simulink model "gm_IP_Core_SS_Switch_and_PWM"  (R2021a)
settings: Solver=VariableStepAuto  StartTime=0.0  StopTime=0.0002  RelTol=1e-3
undefined symbols (not defined in the file or in its folder): f_FPGA_clk, T_FPGA_clk
libraries: hdlmdlgenlib x3, hdlsllib x3
(part 1 of 2)
settings Model: Creator=BHK  LastModifiedBy=hufnagelde
settings SolverCC: AlgebraicLoopSolver=TrustRegion
settings DataIOCC: ReturnWorkspaceOutputs=off
settings OptimizationCC: BlockReduction=off  ConditionallyExecuteInputs=off  DefaultParameterBehavior=Inlined
settings DebuggingCC: AlgebraicLoopMsg=error  InheritedTsInSrcMsg=none  SFMachineParentedDataDiag=warning  ArithmeticOperatorsInVariantConditions=warning
settings HardwareCC: ProdBitPerPointer=32  ProdBitPerSizeT=32  ProdBitPerPtrDiffT=32  ProdLargestAtomicFloat=None  ProdIntDivRoundTo=Undefined  ProdEndianess=Unspecified  ProdWordSize=32  ProdHWDeviceType=ASIC/FPGA->ASIC/FPGA  TargetBitPerLong=64  TargetBitPerPointer=64  TargetBitPerSizeT=64  TargetBitPerPtrDiffT=64  TargetLongLongMode=on  TargetIntDivRoundTo=Zero  TargetEndianess=LittleEndian  TargetWordSize=64  TargetHWDeviceType=Custom Processor->MATLAB Host Computer  ProdEqTarget=off
settings SFSimCC: SimUseLocalCustomCode=off  CustomCodeUndefinedFunction=UseInterfaceOnly
settings RTWCC: RTWUseLocalCustomCode=off

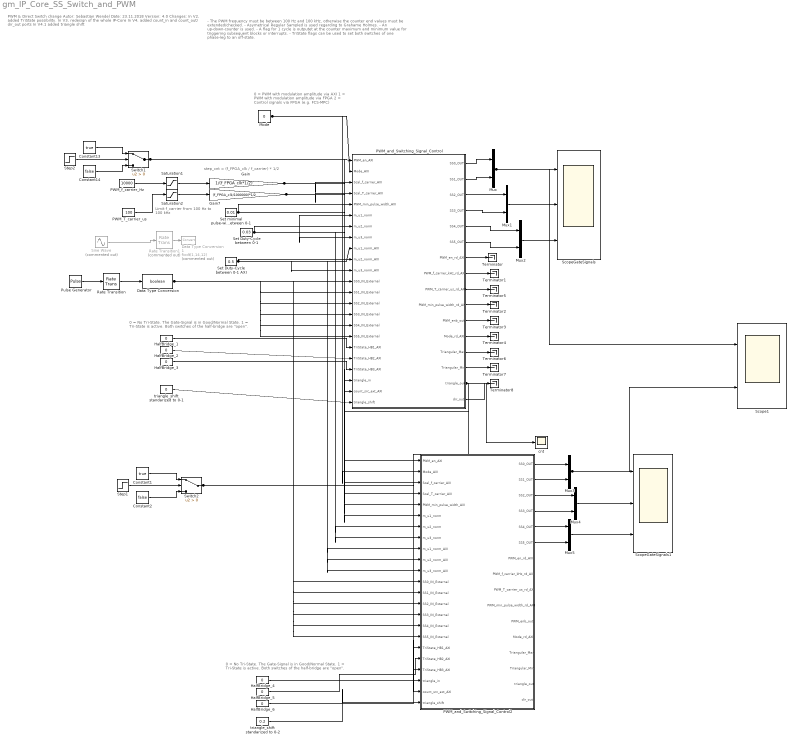
== system gm_IP_Core_SS_Switch_and_PWM ==
  note: 0 = No Tri-State. The Gate-Signal is in Good/Normal State.
      | 1 = Tri-State is active. Both switches of the half-bridge are "open".
  note: - The PWM frequency must be between 100 Hz and 100 kHz, otherwise the counter end values must be extended/checked.
      | - Asymetrical Regular Sampled is used regarding to Grahame Holmes.
      | - An up-down-counter is used.
      | - A flag for 1 cycle is outputet at the counter maximum and minimum value for triggering subsequent blocks or interrupts.
      | - TriState flags can be used to set both switches of one phase-leg to an off-state.
  note: Limit f_carrier from
      | 100 Hz to 100 kHz
  note: step_cnt = (f_FPGA_clk / f_carrier) * 1/2
  note: 0 = PWM with modulation amplitude via AXI
      | 1 = PWM with modulation amplitude via FPGA
      | 2 = Control signals via FPGA (e.g. FCS-MPC)
  note: PWM & Direct Switch change
      |
      | Autor: Sebastian Wendel
      | Date: 23.11.2018
      | Version: 4.0
      | Changes: In V2, added TriState possibility.
      | In V3, redesign of the whole IP-Core
      | In V4, added count_in and count_out/
      | dir_out ports
      | In V4.1 added triangle shift
  note: 0 = No Tri-State. The Gate-Signal is in Good/Normal State.
      | 1 = Tri-State is active. Both switches of the half-bridge are "open".
  Constant1 : Constant  Value=true  SampleTime=T_FPGA_clk
  Constant13 : Constant  Value=true  SampleTime=T_FPGA_clk
  Constant14 : Constant  Value=false  SampleTime=T_FPGA_clk
  Constant2 : Constant  Value=false  SampleTime=T_FPGA_clk
  Data Type Conversion : DataTypeConversion  OutDataTypeStr=boolean
  Data Type Conversion1 : DataTypeConversion  Commented=on  OutDataTypeStr=fixdt(1,14,12)
  Gain : Gain  Gain=1/(f_FPGA_clk*1/2)  OutDataTypeStr=fixdt(0,25,26)
  Gain7 : Gain  Gain=(f_FPGA_clk/1000000)*1/2  OutDataTypeStr=fixdt(0,25,0)
  HalfBridge_{1..6} (6 alike) : Constant  Value=0  OutDataTypeStr=fixdt(0,2,0)  SampleTime=T_FPGA_clk
  Mode : Constant  Value=0  OutDataTypeStr=fixdt(0,2,0)  SampleTime=T_FPGA_clk
  Mux{,1..5} (6 alike) : Mux  Inputs=2
  PWM_T_carrier_us : Constant  Value=100  OutDataTypeStr=uint32  SampleTime=T_FPGA_clk
  PWM_and_Switching_Signal_Control : Subsystem  TreatAsAtomicUnit=on
  PWM_and_Switching_Signal_Control2 : Subsystem  TreatAsAtomicUnit=on
  PWM_f_carrier_Hz : Constant  Value=10000  OutDataTypeStr=uint32  SampleTime=T_FPGA_clk
  Pulse Generator : DiscretePulseGenerator  PulseType=Time based  Period=0.01  PulseWidth=5
  Rate Transition : RateTransition  OutPortSampleTime=T_FPGA_clk
  Rate Transition1 : RateTransition  Commented=on  OutPortSampleTime=T_FPGA_clk
  Saturation1 : Saturate  UpperLimit=100000  LowerLimit=100
  Saturation2 : Saturate  UpperLimit=10000  LowerLimit=10
  Scope1 : Scope  NumInputPorts=2
  ScopeGateSignals : Scope  NumInputPorts=3
  ScopeGateSignals1 : Scope  NumInputPorts=3
  Set Duty-Cycle between 0-1 : Constant  Value=0.03  OutDataTypeStr=fixdt(1,14,12)  SampleTime=T_FPGA_clk
  Set Duty-Cycle between 0-1 AXI : Constant  Value=0.5  OutDataTypeStr=fixdt(1,14,12)  SampleTime=T_FPGA_clk
  Set minimal pulse-width between 0-1 : Constant  Value=0.01  OutDataTypeStr=fixdt(1,18,16)  SampleTime=T_FPGA_clk
  Sine Wave : Sin  Commented=on  Frequency=500  SampleTime=0
  Step1 : Step  Time=0.002  Before=1  SampleTime=T_FPGA_clk
  Step2 : Step  Time=0.002  Before=1  SampleTime=T_FPGA_clk
  Switch1 : Switch  Criteria=u2 > Threshold
  Switch2 : Switch  Criteria=u2 > Threshold
  Terminator{,1..8} (9 alike) : Terminator
  cnt : Scope
  triangle_shift standarized to 0-1 : Constant  Value=0  OutDataTypeStr=fixdt(0,18,17)  SampleTime=T_FPGA_clk
  triangle_shift standarized to 0-2 : Constant  Value=0.2  OutDataTypeStr=fixdt(0,18,17)  SampleTime=T_FPGA_clk
  wires:
  triangle_shift standarized to 0-2/1 -> PWM_and_Switching_Signal_Control2/23(triangle_shift)
  triangle_shift standarized to 0-1/1 -> PWM_and_Switching_Signal_Control/23(triangle_shift)
  Mux4/1 -> ScopeGateSignals1/2
  PWM_and_Switching_Signal_Control2/6(SS5_OUT) -> Mux5/2
  PWM_and_Switching_Signal_Control2/4(SS3_OUT) -> Mux4/2
  PWM_and_Switching_Signal_Control2/3(SS2_OUT) -> Mux4/1
  PWM_and_Switching_Signal_Control2/5(SS4_OUT) -> Mux5/1
  Mux5/1 -> ScopeGateSignals1/3
  Mux3/1 -> Scope1/2, ScopeGateSignals1/1
  PWM_and_Switching_Signal_Control2/2(SS1_OUT) -> Mux3/2
  PWM_and_Switching_Signal_Control2/1(SS0_OUT) -> Mux3/1
  HalfBridge_5/1 -> PWM_and_Switching_Signal_Control2/19(TriState_HB2_AXI)
  HalfBridge_6/1 -> PWM_and_Switching_Signal_Control2/20(TriState_HB3_AXI)
  HalfBridge_4/1 -> PWM_and_Switching_Signal_Control2/18(TriState_HB1_AXI)
  Data Type Conversion/1 -> PWM_and_Switching_Signal_Control/12(SS0_IN_External), PWM_and_Switching_Signal_Control/13(SS1_IN_External), PWM_and_Switching_Signal_Control/14(SS2_IN_External), PWM_and_Switching_Signal_Control/15(SS3_IN_External), PWM_and_Switching_Signal_Control/16(SS4_IN_External), PWM_and_Switching_Signal_Control/17(SS5_IN_External), PWM_and_Switching_Signal_Control2/12(SS0_IN_External), PWM_and_Switching_Signal_Control2/13(SS1_IN_External), PWM_and_Switching_Signal_Control2/15(SS3_IN_External), PWM_and_Switching_Signal_Control2/17(SS5_IN_External), PWM_and_Switching_Signal_Control2/16(SS4_IN_External), PWM_and_Switching_Signal_Control2/14(SS2_IN_External)
  PWM_and_Switching_Signal_Control/15(triangle_out) -> PWM_and_Switching_Signal_Control/21(triangle_in), PWM_and_Switching_Signal_Control2/21(triangle_in), cnt/1
  Switch2/1 -> PWM_and_Switching_Signal_Control/22(count_src_ext_AXI), PWM_and_Switching_Signal_Control2/22(count_src_ext_AXI)
  Constant1/1 -> Switch2/1
  Step1/1 -> Switch2/2
  Constant2/1 -> Switch2/3
  PWM_and_Switching_Signal_Control/16(dir_out) -> Terminator8/1
  Set Duty-Cycle between 0-1/1 -> PWM_and_Switching_Signal_Control2/6(m_u1_norm), PWM_and_Switching_Signal_Control2/7(m_u2_norm), PWM_and_Switching_Signal_Control2/8(m_u3_norm), PWM_and_Switching_Signal_Control/7(m_u2_norm), PWM_and_Switching_Signal_Control/8(m_u3_norm), PWM_and_Switching_Signal_Control/6(m_u1_norm)
  Rate Transition1/1 -> Data Type Conversion1/1
  Saturation2/1 -> Gain7/1
  Saturation1/1 -> Gain/1
  Gain7/1 -> PWM_and_Switching_Signal_Control/4(Scal_T_carrier_AXI), PWM_and_Switching_Signal_Control2/4(Scal_T_carrier_AXI)
  Gain/1 -> PWM_and_Switching_Signal_Control2/3(Scal_f_carrier_AXI), PWM_and_Switching_Signal_Control/3(Scal_f_carrier_AXI)
  PWM_and_Switching_Signal_Control/14(Triangular_Min) -> Terminator7/1
  HalfBridge_1/1 -> PWM_and_Switching_Signal_Control/18(TriState_HB1_AXI)
  HalfBridge_2/1 -> PWM_and_Switching_Signal_Control/19(TriState_HB2_AXI)
  HalfBridge_3/1 -> PWM_and_Switching_Signal_Control/20(TriState_HB3_AXI)
  PWM_and_Switching_Signal_Control/13(Triangular_Max) -> Terminator6/1
  PWM_and_Switching_Signal_Control/9(PWM_T_carrier_us_rd_AXI) -> Terminator5/1
  Pulse Generator/1 -> Rate Transition/1
  Rate Transition/1 -> Data Type Conversion/1
  PWM_T_carrier_us/1 -> Saturation2/1
  Mux1/1 -> ScopeGateSignals/2
  Mux2/1 -> ScopeGateSignals/3
  PWM_and_Switching_Signal_Control/6(SS5_OUT) -> Mux2/2
  PWM_and_Switching_Signal_Control/5(SS4_OUT) -> Mux2/1
  PWM_and_Switching_Signal_Control/4(SS3_OUT) -> Mux1/2
  PWM_and_Switching_Signal_Control/3(SS2_OUT) -> Mux1/1
  Mux/1 -> ScopeGateSignals/1, Scope1/1
  PWM_and_Switching_Signal_Control/2(SS1_OUT) -> Mux/2
  PWM_and_Switching_Signal_Control/1(SS0_OUT) -> Mux/1
  Set Duty-Cycle between 0-1 AXI/1 -> PWM_and_Switching_Signal_Control/9(m_u1_norm_AXI), PWM_and_Switching_Signal_Control/10(m_u2_norm_AXI), PWM_and_Switching_Signal_Control/11(m_u3_norm_AXI), PWM_and_Switching_Signal_Control2/11(m_u3_norm_AXI), PWM_and_Switching_Signal_Control2/10(m_u2_norm_AXI), PWM_and_Switching_Signal_Control2/9(m_u1_norm_AXI)
  PWM_and_Switching_Signal_Control/12(Mode_rd_AXI) -> Terminator4/1
  PWM_and_Switching_Signal_Control/11(PWM_enb_out) -> Terminator3/1
  PWM_and_Switching_Signal_Control/10(PWM_min_pulse_width_rd_AXI) -> Terminator2/1
  PWM_and_Switching_Signal_Control/8(PWM_f_carrier_kHz_rd_AXI) -> Terminator1/1
  PWM_and_Switching_Signal_Control/7(PWM_en_rd_AXI) -> Terminator/1
  Sine Wave/1 -> Rate Transition1/1
  Set minimal pulse-width between 0-1/1 -> PWM_and_Switching_Signal_Control2/5(PWM_min_pulse_width_AXI), PWM_and_Switching_Signal_Control/5(PWM_min_pulse_width_AXI)
  PWM_f_carrier_Hz/1 -> Saturation1/1
  Mode/1 -> PWM_and_Switching_Signal_Control/2(Mode_AXI), PWM_and_Switching_Signal_Control2/2(Mode_AXI)
  Switch1/1 -> PWM_and_Switching_Signal_Control2/1(PWM_en_AXI), PWM_and_Switching_Signal_Control/1(PWM_en_AXI)
  Constant14/1 -> Switch1/3
  Constant13/1 -> Switch1/1
  Step2/1 -> Switch1/2

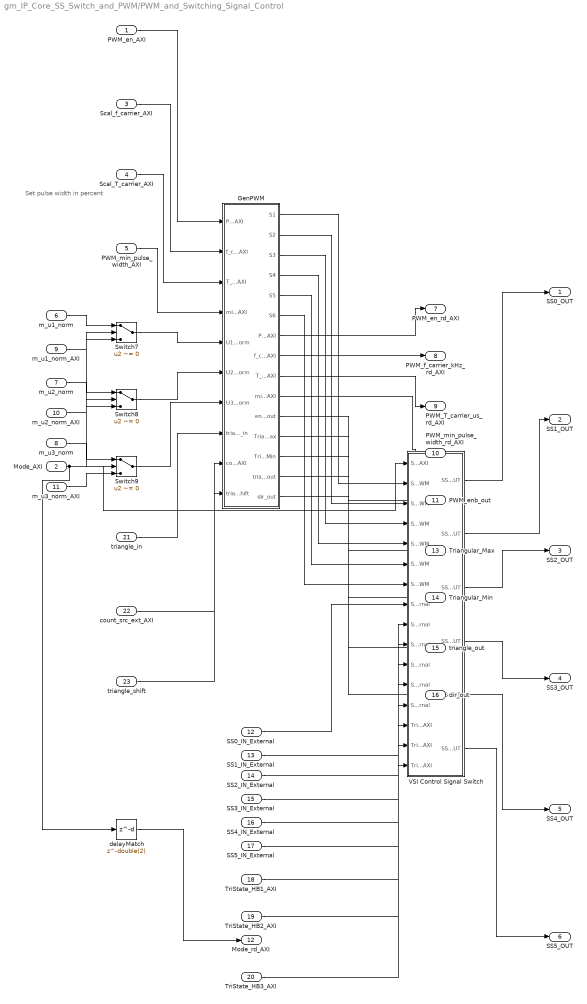
== system gm_IP_Core_SS_Switch_and_PWM/PWM_and_Switching_Signal_Control ==
  note: Set pulse width in percent
  PWM_en_AXI : Inport  OutDataTypeStr=boolean  PortDimensions=1  SampleTime=1e-08
  Mode_AXI : Inport  Port=2  OutDataTypeStr=fixdt(0, 2, 0)  PortDimensions=1  SampleTime=1e-08
  Scal_f_carrier_AXI : Inport  Port=3  OutDataTypeStr=fixdt(0, 25, 26)  PortDimensions=1  SampleTime=1e-08
  Scal_T_carrier_AXI : Inport  Port=4  OutDataTypeStr=fixdt(0, 25, 0)  PortDimensions=1  SampleTime=1e-08
  PWM_min_pulse_width_AXI : Inport  Port=5  OutDataTypeStr=fixdt(1, 18, 16)  PortDimensions=1  SampleTime=1e-08
  m_u1_norm : Inport  Port=6  OutDataTypeStr=fixdt(1, 14, 12)  PortDimensions=1  SampleTime=1e-08
  m_u2_norm : Inport  Port=7  OutDataTypeStr=fixdt(1, 14, 12)  PortDimensions=1  SampleTime=1e-08
  m_u3_norm : Inport  Port=8  OutDataTypeStr=fixdt(1, 14, 12)  PortDimensions=1  SampleTime=1e-08
  m_u1_norm_AXI : Inport  Port=9  OutDataTypeStr=fixdt(1, 14, 12)  PortDimensions=1  SampleTime=1e-08
  m_u2_norm_AXI : Inport  Port=10  OutDataTypeStr=fixdt(1, 14, 12)  PortDimensions=1  SampleTime=1e-08
  m_u3_norm_AXI : Inport  Port=11  OutDataTypeStr=fixdt(1, 14, 12)  PortDimensions=1  SampleTime=1e-08
  SS0_IN_External : Inport  Port=12  OutDataTypeStr=boolean  PortDimensions=1  SampleTime=1e-08
  SS1_IN_External : Inport  Port=13  OutDataTypeStr=boolean  PortDimensions=1  SampleTime=1e-08
  SS2_IN_External : Inport  Port=14  OutDataTypeStr=boolean  PortDimensions=1  SampleTime=1e-08
  SS3_IN_External : Inport  Port=15  OutDataTypeStr=boolean  PortDimensions=1  SampleTime=1e-08
  SS4_IN_External : Inport  Port=16  OutDataTypeStr=boolean  PortDimensions=1  SampleTime=1e-08
  SS5_IN_External : Inport  Port=17  OutDataTypeStr=boolean  PortDimensions=1  SampleTime=1e-08
  TriState_HB1_AXI : Inport  Port=18  OutDataTypeStr=fixdt(0, 2, 0)  PortDimensions=1  SampleTime=1e-08
  TriState_HB2_AXI : Inport  Port=19  OutDataTypeStr=fixdt(0, 2, 0)  PortDimensions=1  SampleTime=1e-08
  TriState_HB3_AXI : Inport  Port=20  OutDataTypeStr=fixdt(0, 2, 0)  PortDimensions=1  SampleTime=1e-08
  triangle_in : Inport  Port=21  OutDataTypeStr=fixdt(0, 18, 17)  PortDimensions=1  SampleTime=1e-08
  count_src_ext_AXI : Inport  Port=22  OutDataTypeStr=boolean  PortDimensions=1  SampleTime=1e-08
  triangle_shift : Inport  Port=23  OutDataTypeStr=fixdt(0, 18, 17)  PortDimensions=1  SampleTime=1e-08
  GenPWM : Subsystem
  Switch7 : Switch  Criteria=u2 ~= 0  Threshold=double(0)  OutDataTypeStr=fixdt(1, 14, 12)  SampleTime=1e-08
  Switch8 : Switch  Criteria=u2 ~= 0  Threshold=double(0)  OutDataTypeStr=fixdt(1, 14, 12)  SampleTime=1e-08
  Switch9 : Switch  Criteria=u2 ~= 0  Threshold=double(0)  OutDataTypeStr=fixdt(1, 14, 12)  SampleTime=1e-08
  VSI Control Signal Switch : Subsystem
  delayMatch : Delay  DelayLength=double(2)  InitialCondition=0  SampleTime=1e-08
  SS0_OUT : Outport  SampleTime=1e-08  VectorParamsAs1DForOutWhenUnconnected=off
  SS1_OUT : Outport  Port=2  SampleTime=1e-08  VectorParamsAs1DForOutWhenUnconnected=off
  SS2_OUT : Outport  Port=3  SampleTime=1e-08  VectorParamsAs1DForOutWhenUnconnected=off
  SS3_OUT : Outport  Port=4  SampleTime=1e-08  VectorParamsAs1DForOutWhenUnconnected=off
  SS4_OUT : Outport  Port=5  SampleTime=1e-08  VectorParamsAs1DForOutWhenUnconnected=off
  SS5_OUT : Outport  Port=6  SampleTime=1e-08  VectorParamsAs1DForOutWhenUnconnected=off
  PWM_en_rd_AXI : Outport  Port=7  SampleTime=1e-08  VectorParamsAs1DForOutWhenUnconnected=off
  PWM_f_carrier_kHz_rd_AXI : Outport  Port=8  SampleTime=1e-08  VectorParamsAs1DForOutWhenUnconnected=off
  PWM_T_carrier_us_rd_AXI : Outport  Port=9  SampleTime=1e-08  VectorParamsAs1DForOutWhenUnconnected=off
  PWM_min_pulse_width_rd_AXI : Outport  Port=10  SampleTime=1e-08  VectorParamsAs1DForOutWhenUnconnected=off
  PWM_enb_out : Outport  Port=11  SampleTime=1e-08  VectorParamsAs1DForOutWhenUnconnected=off
  Mode_rd_AXI : Outport  Port=12  SampleTime=1e-08  VectorParamsAs1DForOutWhenUnconnected=off
  Triangular_Max : Outport  Port=13  SampleTime=1e-08  VectorParamsAs1DForOutWhenUnconnected=off
  Triangular_Min : Outport  Port=14  SampleTime=1e-08  VectorParamsAs1DForOutWhenUnconnected=off
  triangle_out : Outport  Port=15  SampleTime=1e-08  VectorParamsAs1DForOutWhenUnconnected=off
  dir_out : Outport  Port=16  SampleTime=1e-08  VectorParamsAs1DForOutWhenUnconnected=off
  wires:
  PWM_en_AXI/1 -> GenPWM/1(PWM_en_AXI)
  delayMatch/1 -> Mode_rd_AXI/1
  Scal_f_carrier_AXI/1 -> GenPWM/2(f_carrier_kHz_AXI)
  Scal_T_carrier_AXI/1 -> GenPWM/3(T_carrier_us_AXI)
  PWM_min_pulse_width_AXI/1 -> GenPWM/4(min_pulse_width_AXI)
  m_u1_norm/1 -> Switch7/1
  m_u2_norm/1 -> Switch8/1
  m_u3_norm/1 -> Switch9/1
  m_u1_norm_AXI/1 -> Switch7/3
  m_u2_norm_AXI/1 -> Switch8/3
  m_u3_norm_AXI/1 -> Switch9/3
  SS0_IN_External/1 -> VSI Control Signal Switch/8(SS0_IN_External)
  SS1_IN_External/1 -> VSI Control Signal Switch/9(SS1_IN_External)
  SS2_IN_External/1 -> VSI Control Signal Switch/10(SS2_IN_External)
  SS3_IN_External/1 -> VSI Control Signal Switch/11(SS3_IN_External)
  SS4_IN_External/1 -> VSI Control Signal Switch/12(SS4_IN_External)
  SS5_IN_External/1 -> VSI Control Signal Switch/13(SS5_IN_External)
  TriState_HB1_AXI/1 -> VSI Control Signal Switch/14(TriState_HB1_AXI)
  TriState_HB2_AXI/1 -> VSI Control Signal Switch/15(TriState_HB2_AXI)
  TriState_HB3_AXI/1 -> VSI Control Signal Switch/16(TriState_HB3_AXI)
  triangle_in/1 -> GenPWM/8(triangle_in)
  count_src_ext_AXI/1 -> GenPWM/9(count_src_ext_AXI)
  triangle_shift/1 -> GenPWM/10(triangle_shift)
  GenPWM/1(S1) -> VSI Control Signal Switch/2(SS0_IN_PWM)
  GenPWM/2(S2) -> VSI Control Signal Switch/3(SS1_IN_PWM)
  GenPWM/3(S3) -> VSI Control Signal Switch/4(SS2_IN_PWM)
  GenPWM/4(S4) -> VSI Control Signal Switch/5(SS3_IN_PWM)
  GenPWM/5(S5) -> VSI Control Signal Switch/6(SS4_IN_PWM)
  GenPWM/6(S6) -> VSI Control Signal Switch/7(SS5_IN_PWM)
  GenPWM/7(PWM_en_rd_AXI) -> PWM_en_rd_AXI/1
  GenPWM/8(f_carrier_kHz_rd_AXI) -> PWM_f_carrier_kHz_rd_AXI/1
  GenPWM/9(T_carrier_us_rd_AXI) -> PWM_T_carrier_us_rd_AXI/1
  GenPWM/10(min_pulse_width_rd_AXI) -> PWM_min_pulse_width_rd_AXI/1
  GenPWM/11(enb_out) -> PWM_enb_out/1
  GenPWM/12(Triangle_Max) -> Triangular_Max/1
  GenPWM/13(Triangle_Min) -> Triangular_Min/1
  GenPWM/14(triangle_out) -> triangle_out/1
  GenPWM/15(dir_out) -> dir_out/1
  Switch7/1 -> GenPWM/5(U1_norm)
  Switch8/1 -> GenPWM/6(U2_norm)
  Switch9/1 -> GenPWM/7(U3_norm)
  VSI Control Signal Switch/1(SS0_OUT) -> SS0_OUT/1
  VSI Control Signal Switch/2(SS1_OUT) -> SS1_OUT/1
  VSI Control Signal Switch/3(SS2_OUT) -> SS2_OUT/1
  VSI Control Signal Switch/4(SS3_OUT) -> SS3_OUT/1
  VSI Control Signal Switch/5(SS4_OUT) -> SS4_OUT/1
  VSI Control Signal Switch/6(SS5_OUT) -> SS5_OUT/1
  Mode_AXI/1 -> delayMatch/1, Switch9/2, Switch8/2, Switch7/2, VSI Control Signal Switch/1(Switch_AXI)

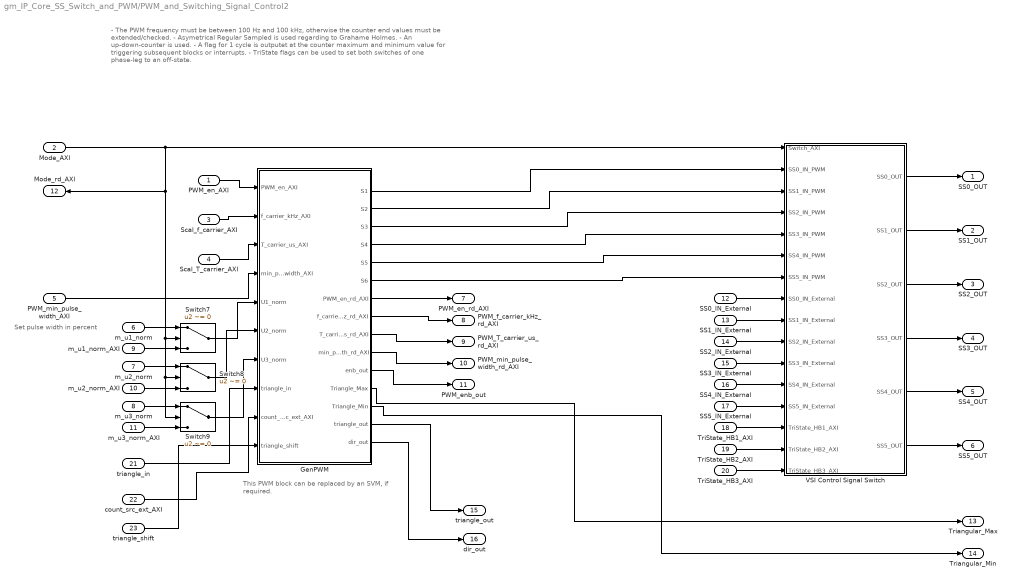
== system gm_IP_Core_SS_Switch_and_PWM/PWM_and_Switching_Signal_Control2 ==
  note: Set pulse width in percent
  note: - The PWM frequency must be between 100 Hz and 100 kHz, otherwise the counter end values must be extended/checked.
      | - Asymetrical Regular Sampled is used regarding to Grahame Holmes.
      | - An up-down-counter is used.
      | - A flag for 1 cycle is outputet at the counter maximum and minimum value for triggering subsequent blocks or interrupts.
      | - TriState flags can be used to set both switches of one phase-leg to an off-state.
  note: This PWM block can be replaced by an SVM,
      | if required.
  PWM_en_AXI : Inport
  Mode_AXI : Inport  Port=2
  Scal_f_carrier_AXI : Inport  Port=3
  Scal_T_carrier_AXI : Inport  Port=4
  PWM_min_pulse_width_AXI : Inport  Port=5
  m_u1_norm : Inport  Port=6
  m_u2_norm : Inport  Port=7
  m_u3_norm : Inport  Port=8
  m_u1_norm_AXI : Inport  Port=9
  m_u2_norm_AXI : Inport  Port=10
  m_u3_norm_AXI : Inport  Port=11
  SS0_IN_External : Inport  Port=12
  SS1_IN_External : Inport  Port=13
  SS2_IN_External : Inport  Port=14
  SS3_IN_External : Inport  Port=15
  SS4_IN_External : Inport  Port=16
  SS5_IN_External : Inport  Port=17
  TriState_HB1_AXI : Inport  Port=18
  TriState_HB2_AXI : Inport  Port=19
  TriState_HB3_AXI : Inport  Port=20
  triangle_in : Inport  Port=21
  count_src_ext_AXI : Inport  Port=22
  triangle_shift : Inport  Port=23
  GenPWM : Subsystem  TreatAsAtomicUnit=on
  Switch7 : Switch  Criteria=u2 ~= 0
  Switch8 : Switch  Criteria=u2 ~= 0
  Switch9 : Switch  Criteria=u2 ~= 0
  VSI Control Signal Switch : Subsystem
  SS0_OUT : Outport  VectorParamsAs1DForOutWhenUnconnected=off
  SS1_OUT : Outport  Port=2  VectorParamsAs1DForOutWhenUnconnected=off
  SS2_OUT : Outport  Port=3  VectorParamsAs1DForOutWhenUnconnected=off
  SS3_OUT : Outport  Port=4  VectorParamsAs1DForOutWhenUnconnected=off
  SS4_OUT : Outport  Port=5  VectorParamsAs1DForOutWhenUnconnected=off
  SS5_OUT : Outport  Port=6  VectorParamsAs1DForOutWhenUnconnected=off
  PWM_en_rd_AXI : Outport  Port=7  VectorParamsAs1DForOutWhenUnconnected=off
  PWM_f_carrier_kHz_rd_AXI : Outport  Port=8  VectorParamsAs1DForOutWhenUnconnected=off
  PWM_T_carrier_us_rd_AXI : Outport  Port=9  VectorParamsAs1DForOutWhenUnconnected=off
  PWM_min_pulse_width_rd_AXI : Outport  Port=10  VectorParamsAs1DForOutWhenUnconnected=off
  PWM_enb_out : Outport  Port=11  VectorParamsAs1DForOutWhenUnconnected=off
  Mode_rd_AXI : Outport  Port=12  VectorParamsAs1DForOutWhenUnconnected=off
  Triangular_Max : Outport  Port=13  VectorParamsAs1DForOutWhenUnconnected=off
  Triangular_Min : Outport  Port=14  VectorParamsAs1DForOutWhenUnconnected=off
  triangle_out : Outport  Port=15  VectorParamsAs1DForOutWhenUnconnected=off
  dir_out : Outport  Port=16  VectorParamsAs1DForOutWhenUnconnected=off
  wires:
  triangle_shift/1 -> GenPWM/10(triangle_shift)
  count_src_ext_AXI/1 -> GenPWM/9(count_src_ext_AXI)
  GenPWM/15(dir_out) -> dir_out/1
  GenPWM/14(triangle_out) -> triangle_out/1
  triangle_in/1 -> GenPWM/8(triangle_in)
  GenPWM/13(Triangle_Min) -> Triangular_Min/1
  TriState_HB3_AXI/1 -> VSI Control Signal Switch/16(TriState_HB3_AXI)
  TriState_HB2_AXI/1 -> VSI Control Signal Switch/15(TriState_HB2_AXI)
  TriState_HB1_AXI/1 -> VSI Control Signal Switch/14(TriState_HB1_AXI)
  GenPWM/12(Triangle_Max) -> Triangular_Max/1
  Scal_T_carrier_AXI/1 -> GenPWM/3(T_carrier_us_AXI)
  Switch7/1 -> GenPWM/5(U1_norm)
  Switch8/1 -> GenPWM/6(U2_norm)
  GenPWM/9(T_carrier_us_rd_AXI) -> PWM_T_carrier_us_rd_AXI/1
  GenPWM/10(min_pulse_width_rd_AXI) -> PWM_min_pulse_width_rd_AXI/1
  GenPWM/8(f_carrier_kHz_rd_AXI) -> PWM_f_carrier_kHz_rd_AXI/1
  GenPWM/7(PWM_en_rd_AXI) -> PWM_en_rd_AXI/1
  m_u3_norm_AXI/1 -> Switch9/3
  m_u3_norm/1 -> Switch9/1
  m_u2_norm_AXI/1 -> Switch8/3
  m_u2_norm/1 -> Switch8/1
  m_u1_norm/1 -> Switch7/1
  m_u1_norm_AXI/1 -> Switch7/3
  Switch9/1 -> GenPWM/7(U3_norm)
  VSI Control Signal Switch/4(SS3_OUT) -> SS3_OUT/1
  SS2_IN_External/1 -> VSI Control Signal Switch/10(SS2_IN_External)
  PWM_min_pulse_width_AXI/1 -> GenPWM/4(min_pulse_width_AXI)
  VSI Control Signal Switch/5(SS4_OUT) -> SS4_OUT/1
  SS5_IN_External/1 -> VSI Control Signal Switch/13(SS5_IN_External)
  PWM_en_AXI/1 -> GenPWM/1(PWM_en_AXI)
  SS4_IN_External/1 -> VSI Control Signal Switch/12(SS4_IN_External)
  VSI Control Signal Switch/2(SS1_OUT) -> SS1_OUT/1
  SS0_IN_External/1 -> VSI Control Signal Switch/8(SS0_IN_External)
  SS3_IN_External/1 -> VSI Control Signal Switch/11(SS3_IN_External)
  VSI Control Signal Switch/3(SS2_OUT) -> SS2_OUT/1
  GenPWM/11(enb_out) -> PWM_enb_out/1
  GenPWM/1(S1) -> VSI Control Signal Switch/2(SS0_IN_PWM)
  VSI Control Signal Switch/6(SS5_OUT) -> SS5_OUT/1
  GenPWM/6(S6) -> VSI Control Signal Switch/7(SS5_IN_PWM)
  GenPWM/5(S5) -> VSI Control Signal Switch/6(SS4_IN_PWM)
  GenPWM/3(S3) -> VSI Control Signal Switch/4(SS2_IN_PWM)
  SS1_IN_External/1 -> VSI Control Signal Switch/9(SS1_IN_External)
  GenPWM/2(S2) -> VSI Control Signal Switch/3(SS1_IN_PWM)
  Scal_f_carrier_AXI/1 -> GenPWM/2(f_carrier_kHz_AXI)
  GenPWM/4(S4) -> VSI Control Signal Switch/5(SS3_IN_PWM)
  Mode_AXI/1 -> VSI Control Signal Switch/1(Switch_AXI), Switch8/2, Switch9/2, Switch7/2, Mode_rd_AXI/1
  VSI Control Signal Switch/1(SS0_OUT) -> SS0_OUT/1

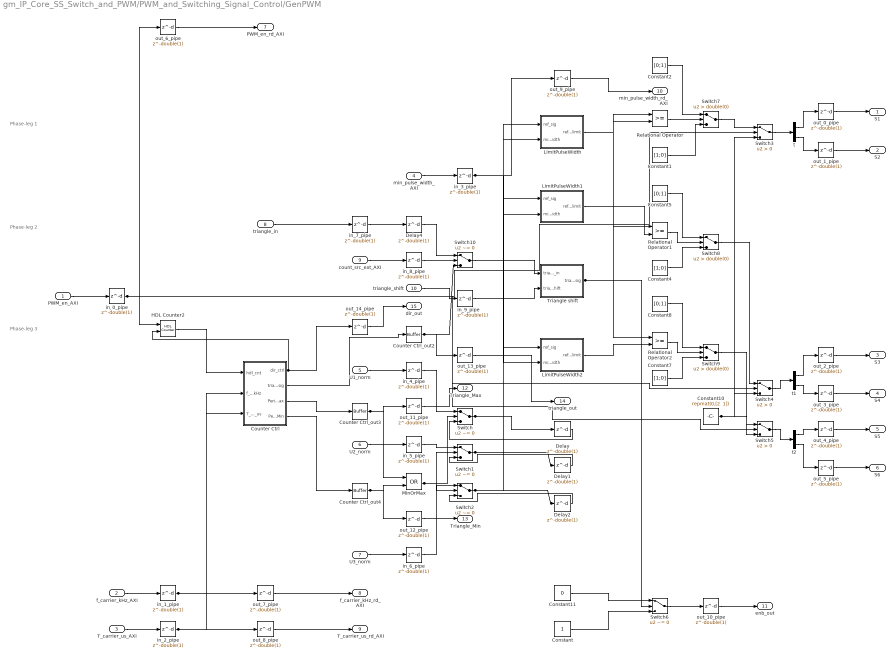
== system gm_IP_Core_SS_Switch_and_PWM/PWM_and_Switching_Signal_Control/GenPWM ==
  note: Phase-leg 3
  note: Phase-leg 2
  note: Phase-leg 1
  PWM_en_AXI : Inport  OutDataTypeStr=boolean  PortDimensions=1  SampleTime=1e-08
  f_carrier_kHz_AXI : Inport  Port=2  OutDataTypeStr=fixdt(0, 25, 26)  PortDimensions=1  SampleTime=1e-08
  T_carrier_us_AXI : Inport  Port=3  OutDataTypeStr=fixdt(0, 25, 0)  PortDimensions=1  SampleTime=1e-08
  min_pulse_width_AXI : Inport  Port=4  OutDataTypeStr=fixdt(1, 18, 16)  PortDimensions=1  SampleTime=1e-08
  U1_norm : Inport  Port=5  OutDataTypeStr=fixdt(1, 14, 12)  PortDimensions=1  SampleTime=1e-08
  U2_norm : Inport  Port=6  OutDataTypeStr=fixdt(1, 14, 12)  PortDimensions=1  SampleTime=1e-08
  U3_norm : Inport  Port=7  OutDataTypeStr=fixdt(1, 14, 12)  PortDimensions=1  SampleTime=1e-08
  triangle_in : Inport  Port=8  OutDataTypeStr=fixdt(0, 18, 17)  PortDimensions=1  SampleTime=1e-08
  count_src_ext_AXI : Inport  Port=9  OutDataTypeStr=boolean  PortDimensions=1  SampleTime=1e-08
  triangle_shift : Inport  Port=10  OutDataTypeStr=fixdt(0, 18, 17)  PortDimensions=1  SampleTime=1e-08
  Constant : Constant  OutDataTypeStr=boolean  SampleTime=1e-08
  Constant1 : Constant  Value=[1;0]  OutDataTypeStr=fixdt(0, 1, 0)  SampleTime=1e-08
  Constant10 : Constant  Value="repmat(0,[2  1])"  OutDataTypeStr=fixdt(0, 1, 0)  SampleTime=1e-08
  Constant11 : Constant  Value=0  OutDataTypeStr=boolean  SampleTime=1e-08
  Constant2 : Constant  Value=[0;1]  OutDataTypeStr=fixdt(0, 1, 0)  SampleTime=1e-08
  Constant4 : Constant  Value=[1;0]  OutDataTypeStr=fixdt(0, 1, 0)  SampleTime=1e-08
  Constant5 : Constant  Value=[0;1]  OutDataTypeStr=fixdt(0, 1, 0)  SampleTime=1e-08
  Constant7 : Constant  Value=[1;0]  OutDataTypeStr=fixdt(0, 1, 0)  SampleTime=1e-08
  Constant8 : Constant  Value=[0;1]  OutDataTypeStr=fixdt(0, 1, 0)  SampleTime=1e-08
  Counter Ctrl : Subsystem
  Counter Ctrl_out2 : hdlmdlgenlib/Buffer
      settings: SourceProductBaseCode=SL
  Counter Ctrl_out3 : hdlmdlgenlib/Buffer
      settings: SourceProductBaseCode=SL
  Counter Ctrl_out4 : hdlmdlgenlib/Buffer
      settings: SourceProductBaseCode=SL
  Delay{,1..2,4} (4 alike) : Delay  DelayLength=double(1)  InitialCondition=0  SampleTime=1e-08
  HDL Counter2 : hdlsllib/Sources/HDL Counter  CountType=Free running  CountInit=double(0)  CountStep=double(1)  CountMax=25  CountFromType=Initial value  CountFrom=double(0)  CountResetPort=off  CountLoadPort=off  CountEnbPort=on  CountDirPort=on  CountHitOutputPort=off  CountDataType=Unsigned  CountWordLen=20  CountFracLen=0  CountSampTime=1e-08
  LimitPulseWidth : Subsystem
  LimitPulseWidth1 : Subsystem
  LimitPulseWidth2 : Subsystem
  MinOrMax : Logic  Operator=OR  AllPortsSameDT=off  OutDataTypeStr=boolean  SampleTime=1e-08
  Relational Operator : RelationalOperator  OutDataTypeStr=boolean  SampleTime=1e-08  RndMeth=Nearest
  Relational Operator1 : RelationalOperator  OutDataTypeStr=boolean  SampleTime=1e-08  RndMeth=Nearest
  Relational Operator2 : RelationalOperator  OutDataTypeStr=boolean  SampleTime=1e-08  RndMeth=Nearest
  Switch : Switch  Criteria=u2 ~= 0  Threshold=double(0)  OutDataTypeStr=fixdt(1, 14, 12)  SampleTime=1e-08
  Switch1 : Switch  Criteria=u2 ~= 0  Threshold=double(0)  OutDataTypeStr=fixdt(1, 14, 12)  SampleTime=1e-08
  Switch10 : Switch  Criteria=u2 ~= 0  Threshold=double(0)  OutDataTypeStr=fixdt(0, 18, 17)  SampleTime=1e-08
  Switch2 : Switch  Criteria=u2 ~= 0  Threshold=double(0)  OutDataTypeStr=fixdt(1, 14, 12)  SampleTime=1e-08
  Switch3 : Switch  Criteria=u2 > Threshold  OutDataTypeStr=fixdt(0, 1, 0)  SampleTime=1e-08
  Switch4 : Switch  Criteria=u2 > Threshold  OutDataTypeStr=fixdt(0, 1, 0)  SampleTime=1e-08
  Switch5 : Switch  Criteria=u2 > Threshold  OutDataTypeStr=fixdt(0, 1, 0)  SampleTime=1e-08
  Switch6 : Switch  Criteria=u2 ~= 0  Threshold=double(0)  OutDataTypeStr=boolean  SampleTime=1e-08
  Switch7 : Switch  Criteria=u2 > Threshold  Threshold=double(0)  OutDataTypeStr=fixdt(0, 1, 0)  SampleTime=1e-08
  Switch8 : Switch  Criteria=u2 > Threshold  Threshold=double(0)  OutDataTypeStr=fixdt(0, 1, 0)  SampleTime=1e-08
  Switch9 : Switch  Criteria=u2 > Threshold  Threshold=double(0)  OutDataTypeStr=fixdt(0, 1, 0)  SampleTime=1e-08
  Triangle shift : Subsystem
  in_0_pipe : Delay  DelayLength=double(1)  InitialCondition=0  SampleTime=1e-08
  in_1_pipe : Delay  DelayLength=double(1)  InitialCondition=0  SampleTime=1e-08
  in_2_pipe : Delay  DelayLength=double(1)  InitialCondition=0  SampleTime=1e-08
  in_3_pipe : Delay  DelayLength=double(1)  InitialCondition=0  SampleTime=1e-08
  in_4_pipe : Delay  DelayLength=double(1)  InitialCondition=0  SampleTime=1e-08
  in_5_pipe : Delay  DelayLength=double(1)  InitialCondition=0  SampleTime=1e-08
  in_6_pipe : Delay  DelayLength=double(1)  InitialCondition=0  SampleTime=1e-08
  in_7_pipe : Delay  DelayLength=double(1)  InitialCondition=0  SampleTime=1e-08
  in_8_pipe : Delay  DelayLength=double(1)  InitialCondition=0  SampleTime=1e-08
  in_9_pipe : Delay  DelayLength=double(1)  InitialCondition=0  SampleTime=1e-08
  out_0_pipe : Delay  DelayLength=double(1)  InitialCondition=0  SampleTime=1e-08
  out_10_pipe : Delay  DelayLength=double(1)  InitialCondition=0  SampleTime=1e-08
  out_11_pipe : Delay  DelayLength=double(1)  InitialCondition=0  SampleTime=1e-08
  out_12_pipe : Delay  DelayLength=double(1)  InitialCondition=0  SampleTime=1e-08
  out_13_pipe : Delay  DelayLength=double(1)  InitialCondition=0  SampleTime=1e-08
  out_14_pipe : Delay  DelayLength=double(1)  InitialCondition=0  SampleTime=1e-08
  out_1_pipe : Delay  DelayLength=double(1)  InitialCondition=0  SampleTime=1e-08
  out_2_pipe : Delay  DelayLength=double(1)  InitialCondition=0  SampleTime=1e-08
  out_3_pipe : Delay  DelayLength=double(1)  InitialCondition=0  SampleTime=1e-08
  out_4_pipe : Delay  DelayLength=double(1)  InitialCondition=0  SampleTime=1e-08
  out_5_pipe : Delay  DelayLength=double(1)  InitialCondition=0  SampleTime=1e-08
  out_6_pipe : Delay  DelayLength=double(1)  InitialCondition=0  SampleTime=1e-08
  out_7_pipe : Delay  DelayLength=double(1)  InitialCondition=0  SampleTime=1e-08
  out_8_pipe : Delay  DelayLength=double(1)  InitialCondition=0  SampleTime=1e-08
  out_9_pipe : Delay  DelayLength=double(1)  InitialCondition=0  SampleTime=1e-08
  t : Demux  Outputs=2
  t1 : Demux  Outputs=2
  t2 : Demux  Outputs=2
  S1 : Outport  SampleTime=1e-08  VectorParamsAs1DForOutWhenUnconnected=off
  S2 : Outport  Port=2  SampleTime=1e-08  VectorParamsAs1DForOutWhenUnconnected=off
  S3 : Outport  Port=3  SampleTime=1e-08  VectorParamsAs1DForOutWhenUnconnected=off
  S4 : Outport  Port=4  SampleTime=1e-08  VectorParamsAs1DForOutWhenUnconnected=off
  S5 : Outport  Port=5  SampleTime=1e-08  VectorParamsAs1DForOutWhenUnconnected=off
  S6 : Outport  Port=6  SampleTime=1e-08  VectorParamsAs1DForOutWhenUnconnected=off
  PWM_en_rd_AXI : Outport  Port=7  SampleTime=1e-08  VectorParamsAs1DForOutWhenUnconnected=off
  f_carrier_kHz_rd_AXI : Outport  Port=8  SampleTime=1e-08  VectorParamsAs1DForOutWhenUnconnected=off
  T_carrier_us_rd_AXI : Outport  Port=9  SampleTime=1e-08  VectorParamsAs1DForOutWhenUnconnected=off
  min_pulse_width_rd_AXI : Outport  Port=10  SampleTime=1e-08  VectorParamsAs1DForOutWhenUnconnected=off
  enb_out : Outport  Port=11  SampleTime=1e-08  VectorParamsAs1DForOutWhenUnconnected=off
  Triangle_Max : Outport  Port=12  SampleTime=1e-08  VectorParamsAs1DForOutWhenUnconnected=off
  Triangle_Min : Outport  Port=13  SampleTime=1e-08  VectorParamsAs1DForOutWhenUnconnected=off
  triangle_out : Outport  Port=14  SampleTime=1e-08  VectorParamsAs1DForOutWhenUnconnected=off
  dir_out : Outport  Port=15  SampleTime=1e-08  VectorParamsAs1DForOutWhenUnconnected=off
  wires:
  in_0_pipe/1 -> Switch5/2, Switch4/2, Switch3/2, out_6_pipe/1, HDL Counter2/1
  in_1_pipe/1 -> out_7_pipe/1, Counter Ctrl/2(f_carrier_kHz)
  in_2_pipe/1 -> out_8_pipe/1, Counter Ctrl/3(T_carrier_us)
  in_3_pipe/1 -> out_9_pipe/1, LimitPulseWidth/2(min_pulse_width), LimitPulseWidth2/2(min_pulse_width), LimitPulseWidth1/2(min_pulse_width)
  in_4_pipe/1 -> Switch/1
  in_5_pipe/1 -> Switch1/1
  in_6_pipe/1 -> Switch2/1
  in_7_pipe/1 -> Delay4/1
  in_8_pipe/1 -> Switch10/2
  in_9_pipe/1 -> Triangle shift/2(triangle_shift)
  Constant/1 -> Switch6/3
  Constant1/1 -> Switch7/3
  Constant10/1 -> Switch5/3, Switch4/3, Switch3/3
  Constant11/1 -> Switch6/1
  Constant2/1 -> Switch7/1
  Constant4/1 -> Switch8/3
  Constant5/1 -> Switch8/1
  Constant7/1 -> Switch9/3
  Constant8/1 -> Switch9/1
  Counter Ctrl_out2/1 -> Switch10/3, out_13_pipe/1
  Counter Ctrl_out3/1 -> MinOrMax/1, out_11_pipe/1
  Counter Ctrl_out4/1 -> MinOrMax/2, out_12_pipe/1
  Delay4/1 -> Switch10/1
  LimitPulseWidth/1(ref_sig_limit) -> Relational Operator/2
  LimitPulseWidth1/1(ref_sig_limit) -> Relational Operator1/2
  LimitPulseWidth2/1(ref_sig_limit) -> Relational Operator2/2
  MinOrMax/1 -> Switch/2, Switch1/2, Switch2/2
  Relational Operator/1 -> Switch7/2
  Relational Operator1/1 -> Switch8/2
  Relational Operator2/1 -> Switch9/2
  Switch10/1 -> Triangle shift/1(triangle_in)
  Switch3/1 -> t/1
  Switch4/1 -> t1/1
  Switch5/1 -> t2/1
  Switch6/1 -> out_10_pipe/1
  Switch7/1 -> Switch3/1
  Switch8/1 -> Switch4/1
  Switch9/1 -> Switch5/1
  Triangle shift/1(triangle_sig) -> Switch6/2, Relational Operator2/1, Relational Operator1/1, Relational Operator/1
  out_0_pipe/1 -> S1/1
  out_1_pipe/1 -> S2/1
  out_2_pipe/1 -> S3/1
  out_3_pipe/1 -> S4/1
  out_4_pipe/1 -> S5/1
  out_5_pipe/1 -> S6/1
  out_6_pipe/1 -> PWM_en_rd_AXI/1
  out_7_pipe/1 -> f_carrier_kHz_rd_AXI/1
  out_8_pipe/1 -> T_carrier_us_rd_AXI/1
  out_9_pipe/1 -> min_pulse_width_rd_AXI/1
  out_10_pipe/1 -> enb_out/1
  out_11_pipe/1 -> Triangle_Max/1
  out_12_pipe/1 -> Triangle_Min/1
  out_13_pipe/1 -> triangle_out/1
  out_14_pipe/1 -> dir_out/1
  t/1 -> out_0_pipe/1
  t/2 -> out_1_pipe/1
  t1/1 -> out_2_pipe/1
  t1/2 -> out_3_pipe/1
  t2/1 -> out_4_pipe/1
  t2/2 -> out_5_pipe/1
  PWM_en_AXI/1 -> in_0_pipe/1
  f_carrier_kHz_AXI/1 -> in_1_pipe/1
  T_carrier_us_AXI/1 -> in_2_pipe/1
  min_pulse_width_AXI/1 -> in_3_pipe/1
  U1_norm/1 -> in_4_pipe/1
  U2_norm/1 -> in_5_pipe/1
  U3_norm/1 -> in_6_pipe/1
  triangle_in/1 -> in_7_pipe/1
  count_src_ext_AXI/1 -> in_8_pipe/1
  triangle_shift/1 -> in_9_pipe/1
  HDL Counter2/1 -> Counter Ctrl/1(hdl_cnt)
  Counter Ctrl/1(dir_ctrl) -> HDL Counter2/2, out_14_pipe/1
  Counter Ctrl/2(triangle_sig) -> Counter Ctrl_out2/1
  Counter Ctrl/3(Period_CenterMax) -> Counter Ctrl_out3/1
  Counter Ctrl/4(Period_CenterMin) -> Counter Ctrl_out4/1
  Delay/1 -> Switch/3
  Switch/1 -> Delay/1, LimitPulseWidth/1(ref_sig)
  Delay1/1 -> Switch1/3
  Switch1/1 -> Delay1/1, LimitPulseWidth1/1(ref_sig)
  Delay2/1 -> Switch2/3
  Switch2/1 -> Delay2/1, LimitPulseWidth2/1(ref_sig)

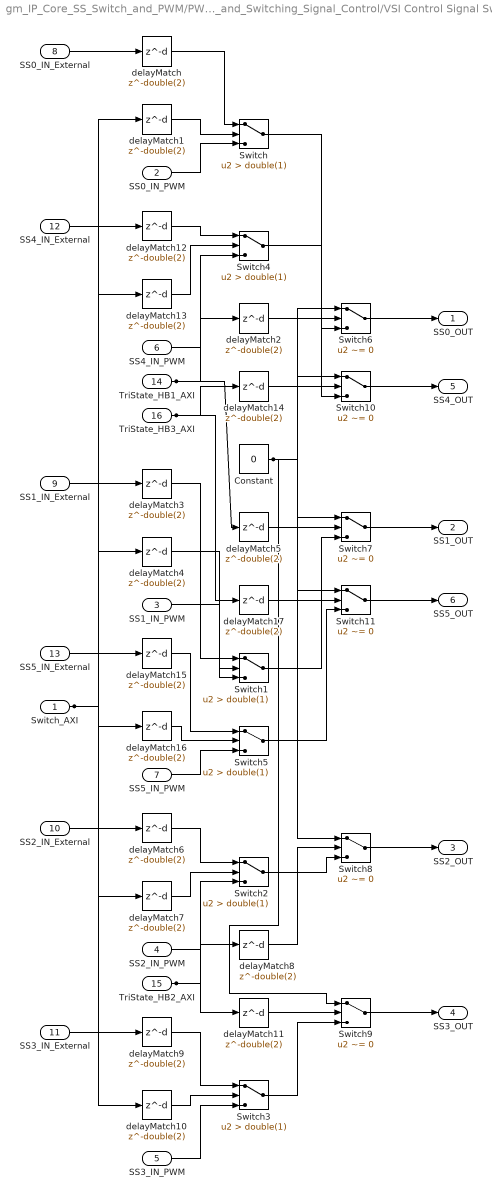
== system gm_IP_Core_SS_Switch_and_PWM/PWM_and_Switching_Signal_Control/VSI Control Signal Switch ==
  Switch_AXI : Inport  OutDataTypeStr=fixdt(0, 2, 0)  PortDimensions=1  SampleTime=1e-08
  SS0_IN_PWM : Inport  Port=2  OutDataTypeStr=fixdt(0, 1, 0)  PortDimensions=1  SampleTime=1e-08
  SS1_IN_PWM : Inport  Port=3  OutDataTypeStr=fixdt(0, 1, 0)  PortDimensions=1  SampleTime=1e-08
  SS2_IN_PWM : Inport  Port=4  OutDataTypeStr=fixdt(0, 1, 0)  PortDimensions=1  SampleTime=1e-08
  SS3_IN_PWM : Inport  Port=5  OutDataTypeStr=fixdt(0, 1, 0)  PortDimensions=1  SampleTime=1e-08
  SS4_IN_PWM : Inport  Port=6  OutDataTypeStr=fixdt(0, 1, 0)  PortDimensions=1  SampleTime=1e-08
  SS5_IN_PWM : Inport  Port=7  OutDataTypeStr=fixdt(0, 1, 0)  PortDimensions=1  SampleTime=1e-08
  SS0_IN_External : Inport  Port=8  OutDataTypeStr=boolean  PortDimensions=1  SampleTime=1e-08
  SS1_IN_External : Inport  Port=9  OutDataTypeStr=boolean  PortDimensions=1  SampleTime=1e-08
  SS2_IN_External : Inport  Port=10  OutDataTypeStr=boolean  PortDimensions=1  SampleTime=1e-08
  SS3_IN_External : Inport  Port=11  OutDataTypeStr=boolean  PortDimensions=1  SampleTime=1e-08
  SS4_IN_External : Inport  Port=12  OutDataTypeStr=boolean  PortDimensions=1  SampleTime=1e-08
  SS5_IN_External : Inport  Port=13  OutDataTypeStr=boolean  PortDimensions=1  SampleTime=1e-08
  TriState_HB1_AXI : Inport  Port=14  OutDataTypeStr=fixdt(0, 2, 0)  PortDimensions=1  SampleTime=1e-08
  TriState_HB2_AXI : Inport  Port=15  OutDataTypeStr=fixdt(0, 2, 0)  PortDimensions=1  SampleTime=1e-08
  TriState_HB3_AXI : Inport  Port=16  OutDataTypeStr=fixdt(0, 2, 0)  PortDimensions=1  SampleTime=1e-08
  Constant : Constant  Value=0  OutDataTypeStr=boolean  SampleTime=1e-08
  Switch{,1..5} (6 alike) : Switch  Criteria=u2 > Threshold  Threshold=double(1)  OutDataTypeStr=boolean  SampleTime=1e-08
  Switch{6..11} (6 alike) : Switch  Criteria=u2 ~= 0  Threshold=double(0)  OutDataTypeStr=boolean  SampleTime=1e-08
  delayMatch{,1..17} (18 alike) : Delay  DelayLength=double(2)  InitialCondition=0  SampleTime=1e-08
  SS0_OUT : Outport  SampleTime=1e-08  VectorParamsAs1DForOutWhenUnconnected=off
  SS1_OUT : Outport  Port=2  SampleTime=1e-08  VectorParamsAs1DForOutWhenUnconnected=off
  SS2_OUT : Outport  Port=3  SampleTime=1e-08  VectorParamsAs1DForOutWhenUnconnected=off
  SS3_OUT : Outport  Port=4  SampleTime=1e-08  VectorParamsAs1DForOutWhenUnconnected=off
  SS4_OUT : Outport  Port=5  SampleTime=1e-08  VectorParamsAs1DForOutWhenUnconnected=off
  SS5_OUT : Outport  Port=6  SampleTime=1e-08  VectorParamsAs1DForOutWhenUnconnected=off
  wires:
  delayMatch1/1 -> Switch/2
  delayMatch/1 -> Switch/1
  delayMatch3/1 -> Switch1/1
  delayMatch6/1 -> Switch2/1
  delayMatch9/1 -> Switch3/1
  delayMatch12/1 -> Switch4/1
  delayMatch15/1 -> Switch5/1
  delayMatch2/1 -> Switch6/2
  delayMatch8/1 -> Switch8/2
  delayMatch14/1 -> Switch10/2
  Constant/1 -> Switch9/1, Switch8/1, Switch7/1, Switch6/1, Switch11/1, Switch10/1
  Switch/1 -> Switch6/3
  Switch1/1 -> Switch7/3
  Switch10/1 -> SS4_OUT/1
  Switch11/1 -> SS5_OUT/1
  Switch2/1 -> Switch8/3
  Switch3/1 -> Switch9/3
  Switch4/1 -> Switch10/3
  Switch5/1 -> Switch11/3
  Switch6/1 -> SS0_OUT/1
  Switch7/1 -> SS1_OUT/1
  Switch8/1 -> SS2_OUT/1
  Switch9/1 -> SS3_OUT/1
  Switch_AXI/1 -> delayMatch16/1, delayMatch13/1, delayMatch10/1, delayMatch7/1, delayMatch4/1, delayMatch1/1
  SS0_IN_PWM/1 -> Switch/3
  SS1_IN_PWM/1 -> Switch1/3
  SS2_IN_PWM/1 -> Switch2/3
  SS3_IN_PWM/1 -> Switch3/3
  SS4_IN_PWM/1 -> Switch4/3
  SS5_IN_PWM/1 -> Switch5/3
  SS0_IN_External/1 -> delayMatch/1
  SS1_IN_External/1 -> delayMatch3/1
  SS2_IN_External/1 -> delayMatch6/1
  SS3_IN_External/1 -> delayMatch9/1
  SS4_IN_External/1 -> delayMatch12/1
  SS5_IN_External/1 -> delayMatch15/1
  TriState_HB1_AXI/1 -> delayMatch5/1, delayMatch2/1
  TriState_HB2_AXI/1 -> delayMatch11/1, delayMatch8/1
  TriState_HB3_AXI/1 -> delayMatch17/1, delayMatch14/1
  delayMatch4/1 -> Switch1/2
  delayMatch5/1 -> Switch7/2
  delayMatch7/1 -> Switch2/2
  delayMatch10/1 -> Switch3/2
  delayMatch11/1 -> Switch9/2
  delayMatch13/1 -> Switch4/2
  delayMatch16/1 -> Switch5/2
  delayMatch17/1 -> Switch11/2

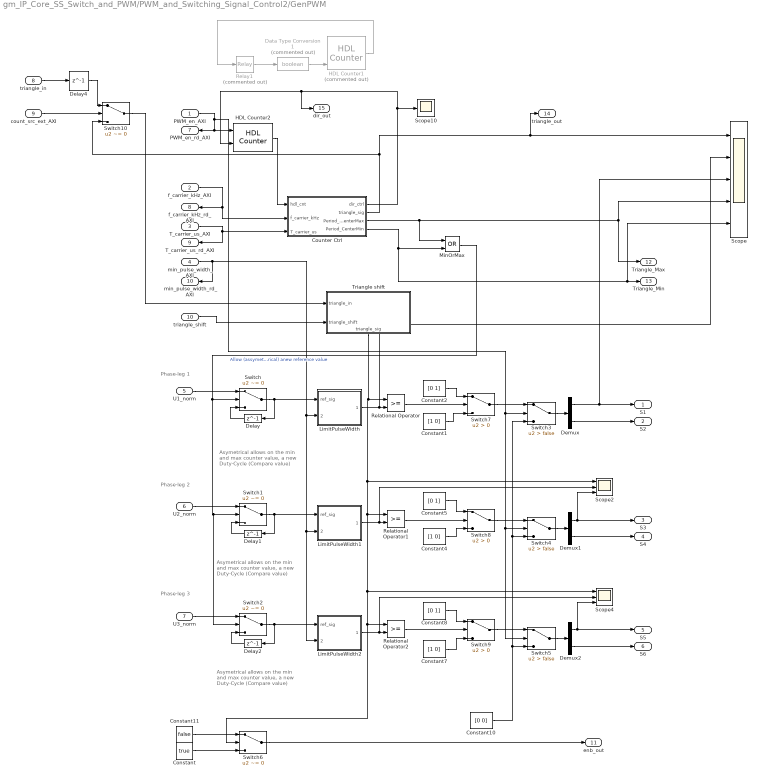
== system gm_IP_Core_SS_Switch_and_PWM/PWM_and_Switching_Signal_Control2/GenPWM ==
  note: Asymetrical allows on the min
      |  and max counter value, a new
      |  Duty-Cycle (Compare value)
  note: Asymetrical allows on the min
      |  and max counter value, a new
      |  Duty-Cycle (Compare value)
  note: Phase-leg 3
  note: Phase-leg 2
  note: Phase-leg 1
  note: Asymetrical allows on the min
      |  and max counter value, a new
      |  Duty-Cycle (Compare value)
  PWM_en_AXI : Inport
  f_carrier_kHz_AXI : Inport  Port=2
  T_carrier_us_AXI : Inport  Port=3
  min_pulse_width_AXI : Inport  Port=4
  U1_norm : Inport  Port=5
  U2_norm : Inport  Port=6
  U3_norm : Inport  Port=7
  triangle_in : Inport  Port=8
  count_src_ext_AXI : Inport  Port=9
  triangle_shift : Inport  Port=10
  Constant : Constant  Value=true  SampleTime=T_FPGA_clk
  Constant1 : Constant  Value=[1 0]  OutDataTypeStr=fixdt(0,1,0)  SampleTime=T_FPGA_clk
  Constant10 : Constant  Value=[0 0]  OutDataTypeStr=fixdt(0,1,0)  SampleTime=T_FPGA_clk
  Constant11 : Constant  Value=false  SampleTime=T_FPGA_clk
  Constant2 : Constant  Value=[0 1]  OutDataTypeStr=fixdt(0,1,0)  SampleTime=T_FPGA_clk
  Constant4 : Constant  Value=[1 0]  OutDataTypeStr=fixdt(0,1,0)  SampleTime=T_FPGA_clk
  Constant5 : Constant  Value=[0 1]  OutDataTypeStr=fixdt(0,1,0)  SampleTime=T_FPGA_clk
  Constant7 : Constant  Value=[1 0]  OutDataTypeStr=fixdt(0,1,0)  SampleTime=T_FPGA_clk
  Constant8 : Constant  Value=[0 1]  OutDataTypeStr=fixdt(0,1,0)  SampleTime=T_FPGA_clk
  Counter Ctrl : Subsystem
  Data Type Conversion1 : DataTypeConversion  Commented=on  OutDataTypeStr=boolean
  Delay{,1..2,4} (4 alike) : Delay  DelayLength=1
  Demux : Demux  Outputs=2
  Demux1 : Demux  Outputs=2
  Demux2 : Demux  Outputs=2
  HDL Counter1 : hdlsllib/Sources/HDL Counter  Commented=on  CountType=Free running  CountInit=0  CountStep=1  CountMax=100  CountFromType=Initial value  CountFrom=0  CountResetPort=on  CountLoadPort=off  CountEnbPort=on  CountDirPort=on  CountHitOutputPort=off  CountDataType=Signed  CountWordLen=8  CountFracLen=0  CountSampTime=Ts
  HDL Counter2 : hdlsllib/Sources/HDL Counter  CountType=Free running  CountInit=0  CountStep=1  CountMax=100  CountFromType=Initial value  CountFrom=0  CountResetPort=off  CountLoadPort=off  CountEnbPort=on  CountDirPort=on  CountHitOutputPort=off  CountDataType=Unsigned  CountWordLen=20  CountFracLen=0  CountSampTime=1
  LimitPulseWidth : Subsystem
  LimitPulseWidth1 : Subsystem
  LimitPulseWidth2 : Subsystem
  MinOrMax : Logic  Operator=OR  AllPortsSameDT=off  OutDataTypeStr=boolean
  Relational Operator : RelationalOperator  OutDataTypeStr=boolean  RndMeth=Nearest
  Relational Operator1 : RelationalOperator  OutDataTypeStr=boolean  RndMeth=Nearest
  Relational Operator2 : RelationalOperator  OutDataTypeStr=boolean  RndMeth=Nearest
  Relay1 : Relay  Commented=on  OnSwitchValue=100  OffSwitchValue=0  OnOutputValue=0  OffOutputValue=1
  Scope : Scope  NumInputPorts=5
  Scope10 : Scope
  Scope2 : Scope  NumInputPorts=3
  Scope4 : Scope  NumInputPorts=3
  Switch : Switch  Criteria=u2 ~= 0  Threshold=1
  Switch1 : Switch  Criteria=u2 ~= 0
  Switch10 : Switch  Criteria=u2 ~= 0  Threshold=1
  Switch2 : Switch  Criteria=u2 ~= 0
  Switch3 : Switch  Criteria=u2 > Threshold  Threshold=false
  Switch4 : Switch  Criteria=u2 > Threshold  Threshold=false
  Switch5 : Switch  Criteria=u2 > Threshold  Threshold=false
  Switch6 : Switch  Criteria=u2 ~= 0
  Switch7 : Switch  Criteria=u2 > Threshold
  Switch8 : Switch  Criteria=u2 > Threshold
  Switch9 : Switch  Criteria=u2 > Threshold
  Triangle shift : Subsystem
      settings: PortSchema="{\"entries\":[{\"content\":{\"sides\":[{\"content\":{\"connectorIds\":[\"In1\",\"In2\"]},\"type\":\"ConnectorPlacement.EquallySpacedRectSide\",\"uuid\":\"31401a1e-1f02-4a04-8b8d-7e372ca2eb91\"},{\"content\":{\"connectorIds\":[],\"side\":\"RIGHT\"},\"type\":\"ConnectorPlacement.EquallySpacedRectSide\",\"uuid\":\"eeacee55-a738-4382-aa93-0b1721e8b59d\"},{\"content\":{\"connectorIds\":[],\"side\":\"TOP\"},\"type\":\"ConnectorPlacement.EquallySpacedRectSide\",\"uuid\":\"464cd606-248c-4fd8-a908-db3c4d4bc914\"},{\"content\":{\"connectorIds\":[\"Out1\"],\"side\":\"BOTTOM\"},\"type\":\"ConnectorPlacement.EquallySpacedRectSide\",\"uuid\":\"cfd70d9c-f1fa-4f72-ba3c-9ec7ae795bff\"}]},\"type\":\"ConnectorPlacement.EquallySpacedConnector\",\"uuid\":\"c5d3fef8-e740-4bdf-a257-7ed33f0852f6\"}],\"packageUris\":[\"http://schema.mathworks.com/mf0/Connector/R2020b\"],\"version\":\"1.0\"}"
  S1 : Outport  VectorParamsAs1DForOutWhenUnconnected=off
  S2 : Outport  Port=2  VectorParamsAs1DForOutWhenUnconnected=off
  S3 : Outport  Port=3  VectorParamsAs1DForOutWhenUnconnected=off
  S4 : Outport  Port=4  VectorParamsAs1DForOutWhenUnconnected=off
  S5 : Outport  Port=5  VectorParamsAs1DForOutWhenUnconnected=off
  S6 : Outport  Port=6  VectorParamsAs1DForOutWhenUnconnected=off
  PWM_en_rd_AXI : Outport  Port=7  VectorParamsAs1DForOutWhenUnconnected=off
  f_carrier_kHz_rd_AXI : Outport  Port=8  VectorParamsAs1DForOutWhenUnconnected=off
  T_carrier_us_rd_AXI : Outport  Port=9  VectorParamsAs1DForOutWhenUnconnected=off
  min_pulse_width_rd_AXI : Outport  Port=10  VectorParamsAs1DForOutWhenUnconnected=off
  enb_out : Outport  Port=11  VectorParamsAs1DForOutWhenUnconnected=off
  Triangle_Max : Outport  Port=12  VectorParamsAs1DForOutWhenUnconnected=off
  Triangle_Min : Outport  Port=13  VectorParamsAs1DForOutWhenUnconnected=off
  triangle_out : Outport  Port=14  VectorParamsAs1DForOutWhenUnconnected=off
  dir_out : Outport  Port=15  VectorParamsAs1DForOutWhenUnconnected=off
  wires:
  Switch10/1 -> Triangle shift/1(triangle_in)
  triangle_shift/1 -> Triangle shift/2(triangle_shift)
  Triangle shift/1(triangle_sig) -> Relational Operator/1, Relational Operator1/1, Relational Operator2/1, Switch6/2, Scope4/1, Scope2/1
  Delay4/1 -> Switch10/1
  HDL Counter2/1 -> Counter Ctrl/1(hdl_cnt)
  count_src_ext_AXI/1 -> Switch10/2
  triangle_in/1 -> Delay4/1
  MinOrMax/1 -> Switch/2, Switch2/2, Switch1/2  "Allow (assymetrical) anew reference value"
  Counter Ctrl/4(Period_CenterMin) -> Triangle_Min/1, Scope/5, MinOrMax/2
  Counter Ctrl/3(Period_CenterMax) -> Scope/4, Triangle_Max/1, MinOrMax/1
  min_pulse_width_AXI/1 -> min_pulse_width_rd_AXI/1, LimitPulseWidth1/2(min_pulse_width), LimitPulseWidth2/2(min_pulse_width), LimitPulseWidth/2(min_pulse_width)
  Switch7/1 -> Switch3/1
  T_carrier_us_AXI/1 -> Counter Ctrl/3(T_carrier_us), T_carrier_us_rd_AXI/1
  Demux2/1 -> S5/1, Scope4/3
  Demux1/1 -> S3/1, Scope2/3
  Constant/1 -> Switch6/3
  Constant11/1 -> Switch6/1
  Switch6/1 -> enb_out/1
  Demux/1 -> S1/1, Scope/3
  Switch2/1 -> Delay2/1, LimitPulseWidth2/1(ref_sig)
  Switch1/1 -> Delay1/1, LimitPulseWidth1/1(ref_sig)
  Switch/1 -> LimitPulseWidth/1(ref_sig), Delay/1
  HDL Counter1/1 -> Relay1/1
  Data Type Conversion1/1 -> HDL Counter1/3
  Relay1/1 -> Data Type Conversion1/1
  f_carrier_kHz_AXI/1 -> Counter Ctrl/2(f_carrier_kHz), f_carrier_kHz_rd_AXI/1
  Counter Ctrl/1(dir_ctrl) -> Scope10/1, HDL Counter2/2, dir_out/1
  U2_norm/1 -> Switch1/1
  U3_norm/1 -> Switch2/1
  U1_norm/1 -> Switch/1
  Constant10/1 -> Switch3/3, Switch4/3, Switch5/3
  Switch3/1 -> Demux/1
  Switch4/1 -> Demux1/1
  Switch8/1 -> Switch4/1
  Switch5/1 -> Demux2/1
  Delay2/1 -> Switch2/3
  Delay1/1 -> Switch1/3
  Delay/1 -> Switch/3
  PWM_en_AXI/1 -> Switch3/2, Switch4/2, Switch5/2, HDL Counter2/1, PWM_en_rd_AXI/1
  Counter Ctrl/2(triangle_sig) -> Switch10/3, Scope/1, triangle_out/1
  LimitPulseWidth2/1(ref_sig_limit) -> Relational Operator2/2, Scope4/2
  LimitPulseWidth1/1(ref_sig_limit) -> Relational Operator1/2, Scope2/2
  LimitPulseWidth/1(ref_sig_limit) -> Relational Operator/2, Scope/2
  Constant2/1 -> Switch7/1
  Constant1/1 -> Switch7/3
  Constant4/1 -> Switch8/3
  Relational Operator1/1 -> Switch8/2
  Constant5/1 -> Switch8/1
  Demux1/2 -> S4/1
  Relational Operator/1 -> Switch7/2
  Demux/2 -> S2/1
  Switch9/1 -> Switch5/1
  Relational Operator2/1 -> Switch9/2
  Constant8/1 -> Switch9/1
  Demux2/2 -> S6/1
  Constant7/1 -> Switch9/3

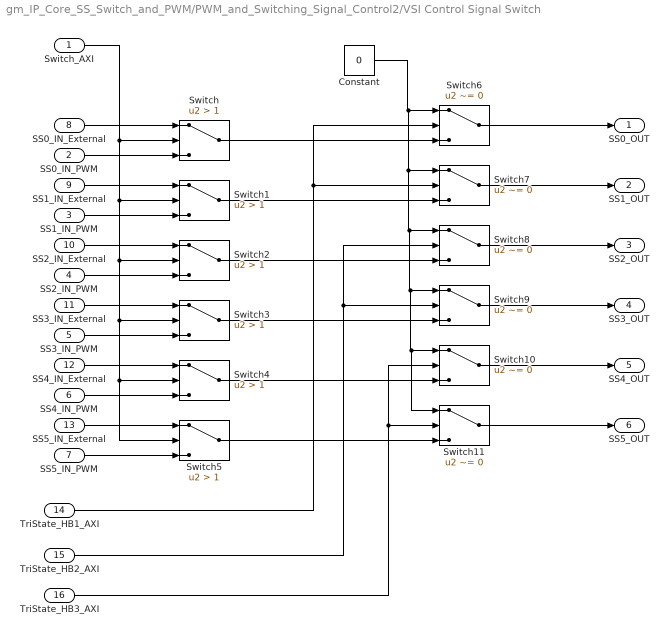
== system gm_IP_Core_SS_Switch_and_PWM/PWM_and_Switching_Signal_Control2/VSI Control Signal Switch ==
  Switch_AXI : Inport
  SS0_IN_PWM : Inport  Port=2
  SS1_IN_PWM : Inport  Port=3
  SS2_IN_PWM : Inport  Port=4
  SS3_IN_PWM : Inport  Port=5
  SS4_IN_PWM : Inport  Port=6
  SS5_IN_PWM : Inport  Port=7
  SS0_IN_External : Inport  Port=8
  SS1_IN_External : Inport  Port=9
  SS2_IN_External : Inport  Port=10
  SS3_IN_External : Inport  Port=11
  SS4_IN_External : Inport  Port=12
  SS5_IN_External : Inport  Port=13
  TriState_HB1_AXI : Inport  Port=14
  TriState_HB2_AXI : Inport  Port=15
  TriState_HB3_AXI : Inport  Port=16
  Constant : Constant  Value=0  OutDataTypeStr=boolean  SampleTime=T_FPGA_clk
  Switch{,1..5} (6 alike) : Switch  Criteria=u2 > Threshold  Threshold=1
  Switch{6..11} (6 alike) : Switch  Criteria=u2 ~= 0  Threshold=1
  SS0_OUT : Outport  VectorParamsAs1DForOutWhenUnconnected=off
  SS1_OUT : Outport  Port=2  VectorParamsAs1DForOutWhenUnconnected=off
  SS2_OUT : Outport  Port=3  VectorParamsAs1DForOutWhenUnconnected=off
  SS3_OUT : Outport  Port=4  VectorParamsAs1DForOutWhenUnconnected=off
  SS4_OUT : Outport  Port=5  VectorParamsAs1DForOutWhenUnconnected=off
  SS5_OUT : Outport  Port=6  VectorParamsAs1DForOutWhenUnconnected=off
  wires:
  Constant/1 -> Switch6/1, Switch7/1, Switch8/1, Switch9/1, Switch10/1, Switch11/1
  Switch6/1 -> SS0_OUT/1
  Switch7/1 -> SS1_OUT/1
  Switch8/1 -> SS2_OUT/1
  Switch9/1 -> SS3_OUT/1
  Switch10/1 -> SS4_OUT/1
  Switch11/1 -> SS5_OUT/1
  TriState_HB1_AXI/1 -> Switch7/2, Switch6/2
  TriState_HB2_AXI/1 -> Switch9/2, Switch8/2
  TriState_HB3_AXI/1 -> Switch11/2, Switch10/2
  SS5_IN_PWM/1 -> Switch5/3
  SS5_IN_External/1 -> Switch5/1
  SS4_IN_PWM/1 -> Switch4/3
  SS4_IN_External/1 -> Switch4/1
  SS3_IN_PWM/1 -> Switch3/3
  SS3_IN_External/1 -> Switch3/1
  SS2_IN_PWM/1 -> Switch2/3
  SS2_IN_External/1 -> Switch2/1
  SS1_IN_PWM/1 -> Switch1/3
  SS1_IN_External/1 -> Switch1/1
  SS0_IN_External/1 -> Switch/1
  SS0_IN_PWM/1 -> Switch/3
  Switch4/1 -> Switch10/3
  Switch1/1 -> Switch7/3
  Switch2/1 -> Switch8/3
  Switch3/1 -> Switch9/3
  Switch/1 -> Switch6/3
  Switch5/1 -> Switch11/3
  Switch_AXI/1 -> Switch/2, Switch1/2, Switch2/2, Switch3/2, Switch5/2, Switch4/2
